simulink model "Project_UR5"  (Simulink 8.3)
settings: Solver=ode3  StartTime=0.0  StopTime=tf  FixedStep=ts  RelTol=1e-3
values from neighbouring files (symbols this model uses):
  qi = [0;pi/4;0;-pi/3;0;0]    [initial.m]
(part 1 of 3)
settings Model: Creator=H3  LastModifiedBy=AMIN
settings DataIOCC: SignalLoggingSaveFormat=Dataset
settings DebuggingCC: UnderspecifiedInitializationDetection=Simplified  StateNameClashWarn=none
settings GRTTargetCC: CombineOutputUpdateFcns=on  GRTInterface=off

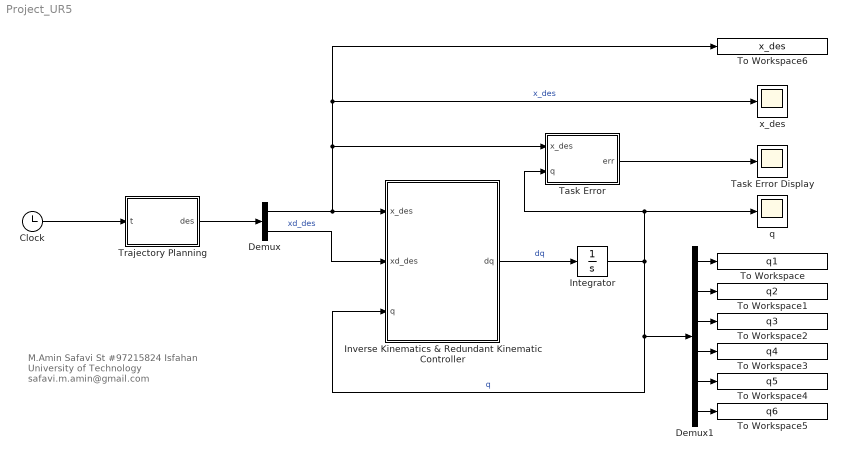
== system Project_UR5 ==
  note: M.Amin Safavi
      | St #97215824
      | Isfahan University of Technology
      | safavi.m.amin@gmail.com
  " Task Error" : MATLAB Function  TreatAsAtomicUnit=on
  " To Workspace6" : ToWorkspace  VariableName=x_des  SampleTime=-1
  Clock : Clock
  Demux : Demux  Outputs=2
  Demux1 : Demux  Outputs=6
  Integrator : Integrator  InitialCondition=qi
  Inverse Kinematics & Redundant Kinematic Controller : MATLAB Function  TreatAsAtomicUnit=on
  Task Error Display : Scope
  To Workspace : ToWorkspace  VariableName=q1  SampleTime=-1
  To Workspace1 : ToWorkspace  VariableName=q2  SampleTime=-1
  To Workspace2 : ToWorkspace  VariableName=q3  SampleTime=-1
  To Workspace3 : ToWorkspace  VariableName=q4  SampleTime=-1
  To Workspace4 : ToWorkspace  VariableName=q5  SampleTime=-1
  To Workspace5 : ToWorkspace  VariableName=q6  SampleTime=-1
  Trajectory Planning : MATLAB Function  TreatAsAtomicUnit=on
  "q " : Scope
      settings: SaveName=ScopeData2
  x_des : Scope
  wires:
  Clock/1 -> Trajectory Planning/1(t)
  Trajectory Planning/1(des) -> Demux/1
  Demux/1 -> " To Workspace6"/1, x_des/1, " Task Error"/1(x_des), Inverse Kinematics & Redundant Kinematic Controller/1(x_des)  "x_des"
  Demux/2 -> Inverse Kinematics & Redundant Kinematic Controller/2(xd_des)  "xd_des"
  Inverse Kinematics & Redundant Kinematic Controller/1(dq) -> Integrator/1  "dq"
  Integrator/1 -> Inverse Kinematics & Redundant Kinematic Controller/3(q), Demux1/1, " Task Error"/2(q), "q "/1  "q"
  Demux1/1 -> To Workspace/1
  Demux1/2 -> To Workspace1/1
  Demux1/3 -> To Workspace2/1
  Demux1/4 -> To Workspace3/1
  Demux1/5 -> To Workspace4/1
  Demux1/6 -> To Workspace5/1
  " Task Error"/1(err) -> Task Error Display/1
